simulink model "exnb4137986_Q9"  (R2024b)
settings: Solver=VariableStepAuto  StartTime=0.0  StopTime=10.0  RelTol=1e-3
values from neighbouring files (symbols this model uses):
  K = place(A, B, lambda_cl)    [exnb4137986_Q6_par.m]    (also in exnb4137986_Q8_par.m; exnb4137986_Q9_par.m)
  m_star_1 = double(subs(m, x2, omega_star_1))    [exnb4137986_Q4_par.m]    (also in exnb4137986_Q6_par.m; exnb4137986_Q8_par.m; exnb4137986_Q9_par.m)
  m_star_2 = double(subs(m, x2, omega_star_2))    [exnb4137986_Q4_par.m]    (also in exnb4137986_Q6_par.m; exnb4137986_Q8_par.m; exnb4137986_Q9_par.m)
  omega_star_1 = 200    [exnb4137986_Q4_par.m]    (also in exnb4137986_Q6_par.m; exnb4137986_Q8_par.m; exnb4137986_Q9_par.m)
  omega_star_2 = 300    [exnb4137986_Q4_par.m]    (also in exnb4137986_Q6_par.m; exnb4137986_Q8_par.m; exnb4137986_Q9_par.m)
  r = 300    [exnb4137986_Q8_par.m]    (also in exnb4137986_Q9_par.m)
  u_star_1 = double(subs(u, x2, omega_star_1))    [exnb4137986_Q4_par.m]    (also in exnb4137986_Q6_par.m; exnb4137986_Q8_par.m; exnb4137986_Q9_par.m)
  values = [1, 10, 0.1, 40]    [exnb4137986_Q4_par.m]    (also in exnb4137986_Q6_par.m; exnb4137986_Q8_par.m; exnb4137986_Q9_par.m)
undefined symbols (not defined in the file or in its folder): a_vect, alpha_vect
settings Model: Creator=therkelsen  LastModifiedBy=therkelsen

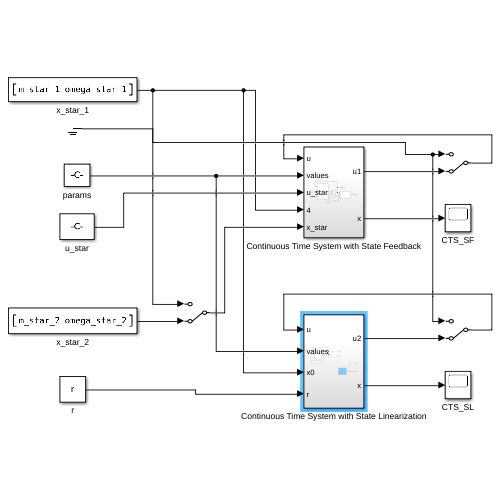
[thumbnail: Simulink's stored preview of the top-level diagram]
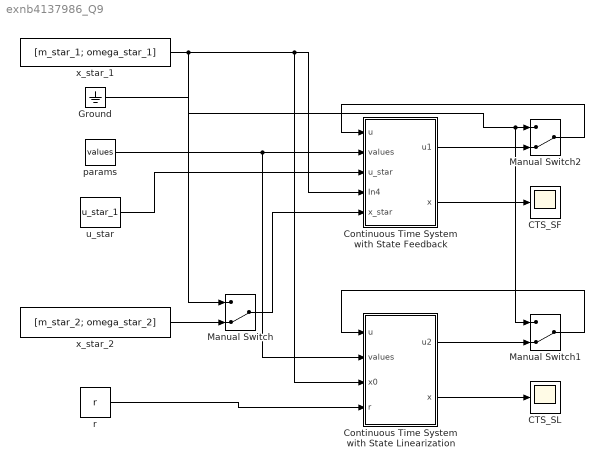
== system exnb4137986_Q9 ==
  CTS_SF : Scope
  CTS_SL : Scope
  Continuous Time System with State Feedback : Subsystem
  Continuous Time System with State Linearization : Subsystem
  Ground : Ground
  Manual Switch : ManualSwitch  CurrentSetting=0
  Manual Switch1 : ManualSwitch  CurrentSetting=0
  Manual Switch2 : ManualSwitch  CurrentSetting=0
  params : Constant  Value=values
  r : Constant  Value=r
  u_star : Constant  Value=u_star_1
  x_star_1 : Constant  Value=[m_star_1; omega_star_1]
  x_star_2 : Constant  Value=[m_star_2; omega_star_2]
  wires:
  x_star_2/1 -> Manual Switch/2
  Continuous Time System with State Feedback/2(x) -> CTS_SF/1
  Continuous Time System with State Feedback/1(u1) -> Manual Switch2/2
  r/1 -> Continuous Time System with State Linearization/4(r)
  params/1 -> Continuous Time System with State Linearization/2(values), Continuous Time System with State Feedback/2(values)
  Ground/1 -> Manual Switch1/1, Manual Switch2/1
  Manual Switch/1 -> Continuous Time System with State Feedback/5(x_star)
  u_star/1 -> Continuous Time System with State Feedback/3(u_star)
  Manual Switch2/1 -> Continuous Time System with State Feedback/1(u)
  Continuous Time System with State Linearization/2(x) -> CTS_SL/1
  Manual Switch1/1 -> Continuous Time System with State Linearization/1(u)
  x_star_1/1 -> Continuous Time System with State Linearization/3(x0), Continuous Time System with State Feedback/4(In4), Manual Switch/1
  Continuous Time System with State Linearization/1(u2) -> Manual Switch1/2

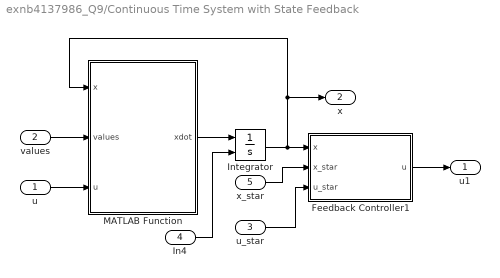
== system exnb4137986_Q9/Continuous Time System with State Feedback ==
  u : Inport
  values : Inport  Port=2
  u_star : Inport  Port=3
  In4 : Inport  Port=4
  x_star : Inport  Port=5
  Feedback Controller1 : Subsystem
  Integrator : Integrator  InitialConditionSource=external
  MATLAB Function : MATLAB Function  TreatAsAtomicUnit=on
  u1 : Outport
  x : Outport  Port=2
  wires:
  Feedback Controller1/1(u) -> u1/1
  Integrator/1 -> x/1, MATLAB Function/1(x), Feedback Controller1/1(x)
  In4/1 -> Integrator/2
  u_star/1 -> Feedback Controller1/3(u_star)
  x_star/1 -> Feedback Controller1/2(x_star)
  MATLAB Function/1(xdot) -> Integrator/1
  u/1 -> MATLAB Function/3(u)
  values/1 -> MATLAB Function/2(values)

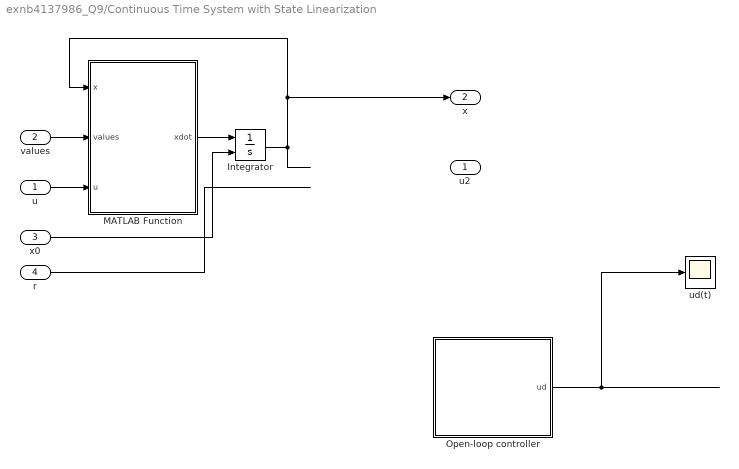
== system exnb4137986_Q9/Continuous Time System with State Linearization ==
  u : Inport
  values : Inport  Port=2
  x0 : Inport  Port=3
  r : Inport  Port=4
  Integrator : Integrator  InitialConditionSource=external
  MATLAB Function : MATLAB Function  TreatAsAtomicUnit=on
  Open-loop controller : Subsystem
  ud(t) : Scope
  u2 : Outport
  x : Outport  Port=2
  wires:
  ? -> u2/1
  Integrator/1 -> x/1, MATLAB Function/1(x)
  x0/1 -> Integrator/2
  MATLAB Function/1(xdot) -> Integrator/1
  u/1 -> MATLAB Function/3(u)
  values/1 -> MATLAB Function/2(values)
  r/1 -> ?
  Open-loop controller/1(ud) -> ud(t)/1

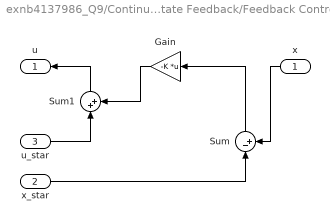
== system exnb4137986_Q9/Continuous Time System with State Feedback/Feedback Controller1 ==
  x : Inport
  x_star : Inport  Port=2
  u_star : Inport  Port=3
  Gain : Gain  Gain=-K  Multiplication=Matrix(K*u)
  Sum : Sum  Inputs=|-+
  Sum1 : Sum  Inputs=|++
  u : Outport
  wires:
  x/1 -> Sum/2
  Gain/1 -> Sum1/2
  Sum/1 -> Gain/1
  x_star/1 -> Sum/1
  u_star/1 -> Sum1/1
  Sum1/1 -> u/1

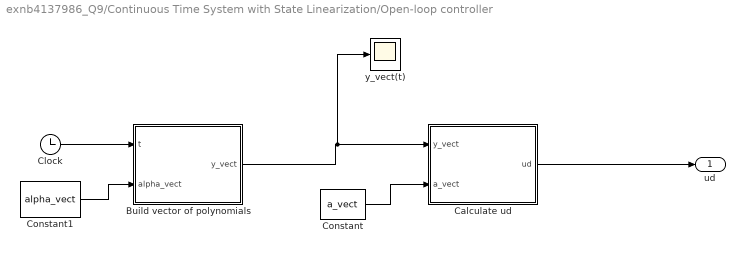
== system exnb4137986_Q9/Continuous Time System with State Linearization/Open-loop controller ==
  Build vector of polynomials : MATLAB Function  TreatAsAtomicUnit=on
  Calculate ud : MATLAB Function  TreatAsAtomicUnit=on
  Clock : Clock
  Constant : Constant  Value=a_vect  VectorParams1D=off
  Constant1 : Constant  Value=alpha_vect  VectorParams1D=off
  y_vect(t) : Scope
  ud : Outport
  wires:
  Build vector of polynomials/1(y_vect) -> y_vect(t)/1, Calculate ud/1(y_vect)
  Constant/1 -> Calculate ud/2(a_vect)
  Constant1/1 -> Build vector of polynomials/2(alpha_vect)
  Clock/1 -> Build vector of polynomials/1(t)
  Calculate ud/1(ud) -> ud/1

== matlab function exnb4137986_Q9/Continuous Time System with State Feedback/MATLAB Function ==
  data: x input; values input; u input; xdot output
function xdot = fcn(x, values, u)

q1 = values(1);
q2 = values(2);
q3 = values(3);
J = values(4);

xdot = [-q1*x(2)*x(1) + u;
         q2/J*x(1) - q3/J*x(2)];

== matlab function exnb4137986_Q9/Continuous Time System with State Linearization/Open-loop controller/Build vector of polynomials ==
  data: t input; y_vect output; alpha_vect input
function y_vect = fcn(t,alpha_vect)


t_vect0 = [ 1 ; t ; t^2 ; t^3 ; t^4 ; t^5 ]; % vector of t values
t_vect1 = [ 0 ; 1 ; 2*t ; 3*t^2 ; 4*t^3 ; 5*t^4 ]; % derivative of t_vect0
t_vect2 = [ 0 ; 0 ; 2 ; 2*3*t ; 3*4*t^2 ; 4*5*t^3 ]; % derivative of t_vect1
t_vect3 = [ 0 ; 0 ; 0 ; 2*3 ; 2*3*4*t ; 3*4*5*t^2 ]; % derivative of t_vect2



yd = t_vect0'*alpha_vect;
yd_dot = t_vect1'*alpha_vect;
yd_ddot = t_vect2'*alpha_vect;
yd_3dot = t_vect3'*alpha_vect;

y_vect = [ yd ; yd_dot ; yd_ddot ; yd_3dot ];

== matlab function exnb4137986_Q9/Continuous Time System with State Linearization/Open-loop controller/Calculate ud ==
  data: y_vect input; ud output; a_vect input
function ud = fcn(y_vect,a_vect)

ae_vect = [ a_vect ; 1 ];


% computation open-loop input
ud = ae_vect' * y_vect;

== matlab function exnb4137986_Q9/Continuous Time System with State Linearization/MATLAB Function ==
  data: x input; values input; u input; xdot output
function xdot = fcn(x, values, u)

q1 = values(1);
q2 = values(2);
q3 = values(3);
J = values(4);

xdot = [-q1*x(2)*x(1) + u;
         q2/J*x(1) - q3/J*x(2)];
